simulink model "xpcpid"  (Simulink 7.3)
settings: Solver=FixedStepDiscrete  StartTime=0.0  StopTime=10000  FixedStep=Ts  RelTol=1e-3
values from neighbouring files (symbols this model uses):
  K = 3.86    [Copy_of_benchmark.m]    (also in benchmark.m = 17.85; setpidparam.m = 1)
  mu = 0.1    [Copy_of_benchmark.m]    (also in benchmark.m; setpidparam.m)
  N = 4    [Copy_of_benchmark.m]    (also in benchmark.m = 2; setpidparam.m = 2)
  Td = 0    [Copy_of_benchmark.m]    (also in benchmark.m = 0.2983; setpidparam.m = 0.1)
  theta = [anti_wind_up; anti_bump; Kf]    [Copy_of_benchmark.m]    (also in benchmark.m = [0]; setpidparam.m = 10)
  Ti = 27    [Copy_of_benchmark.m]    (also in benchmark.m = 1.1932; setpidparam.m = 10)
  Ts = 0.02    [Copy_of_benchmark.m]    (also in benchmark.m; setpidparam.m)
  u0 = 4    [Copy_of_benchmark.m]    (also in setpidparam.m = 0)
  ubounds = [0;10]    [Copy_of_benchmark.m]    (also in benchmark.m = [-6;6]; setpidparam.m = [-4;6])
  y0 = 5.5    [Copy_of_benchmark.m]    (also in setpidparam.m = 0)
libraries: xpclib x4, xpcnilib x2
settings Model: Creator=andrecb  LastModifiedBy=petersson  SimulationMode=external  ExtModeTrigDuration=100  BufferReuse=off
settings OptimizationCC: BlockReduction=off  OptimizeBlockIOStorage=off  BufferReuse=off  ExpressionFolding=off  LocalBlockOutputs=off
settings HardwareCC: ProdIntDivRoundTo=Zero  ProdEndianess=LittleEndian  ProdHWDeviceType=Generic->32-bit x86 compatible
settings RTWCC: SystemTargetFile=xpctarget.tlc  TemplateMakefile=xpc_default_tmf  Description=xPC Target  RTWVerbose=off  ProcessScript=xpctarget_make_rtw_hook  RTWCompilerOptimization=On
settings xpcTargetCC: TargetFcnLib=ansi_tfl_table_tmw.mat  TargetFunctionLibrary=ANSI_C  ParMdlRefBuildCompliant=off  PortableWordSizes=off

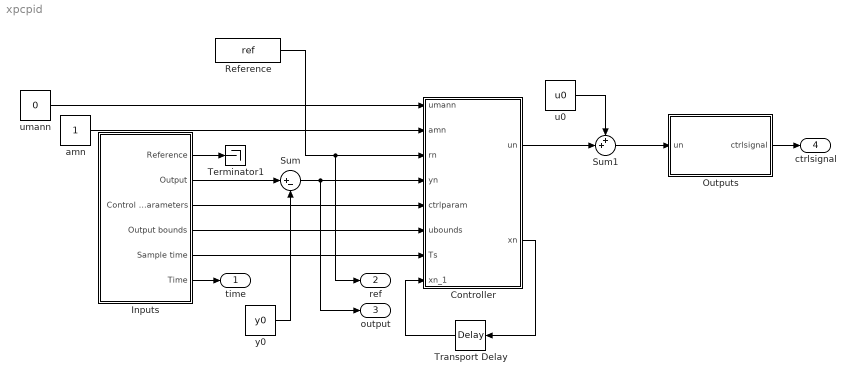
== system xpcpid ==
  Controller : Stateflow chart
  Inputs : Subsystem
  Outputs : Subsystem
  Reference : FromWorkspace  VariableName=ref  SampleTime=Ts
  Sum : Sum  Inputs=|+-  OutDataType=fixdt(1, 16)  OutScaling=2^0
  Sum1 : Sum  Inputs=++|  OutDataType=fixdt(1, 16)  OutScaling=2^0
  Terminator1 : Terminator
  Transport Delay : TransportDelay  DelayTime=Ts  InitialOutput=zeros(N,1)  FixedBuffer=on
  amn : Constant  OutDataType=fixdt(1, 16)  OutScaling=2^0
  u0 : Constant  Value=u0  OutDataType=fixdt(1, 16)  OutScaling=2^0  SampleTime=Ts
  umann : Constant  Value=0  OutDataType=fixdt(1, 16)  OutScaling=2^0
  y0 : Constant  Value=y0  OutDataType=fixdt(1, 16)  OutScaling=2^0  SampleTime=Ts
  time : Outport  SampleTime=Ts  OutDataType=fixdt(1, 16)  OutScaling=2^0
  ref : Outport  Port=2  SampleTime=Ts  OutDataType=fixdt(1, 16)  OutScaling=2^0
  output : Outport  Port=3  SampleTime=Ts  OutDataType=fixdt(1, 16)  OutScaling=2^0
  ctrlsignal : Outport  Port=4  SampleTime=Ts  OutDataType=fixdt(1, 16)  OutScaling=2^0
  wires:
  umann/1 -> Controller/1(umann)
  amn/1 -> Controller/2(amn)
  Inputs/3(Control parameters) -> Controller/5(ctrlparam)
  Controller/2(xn) -> Transport Delay/1
  Transport Delay/1 -> Controller/8(xn_1)
  Inputs/4(Output bounds) -> Controller/6(ubounds)
  Inputs/5(Sample time) -> Controller/7(Ts)
  Inputs/6(Time) -> time/1
  Outputs/1(ctrlsignal) -> ctrlsignal/1
  Controller/1(un) -> Sum1/2
  u0/1 -> Sum1/1
  Sum/1 -> Controller/4(yn), output/1
  Inputs/2(Output) -> Sum/1
  y0/1 -> Sum/2
  Inputs/1(Reference) -> Terminator1/1
  Reference/1 -> ref/1, Controller/3(rn)
  Sum1/1 -> Outputs/1(un)

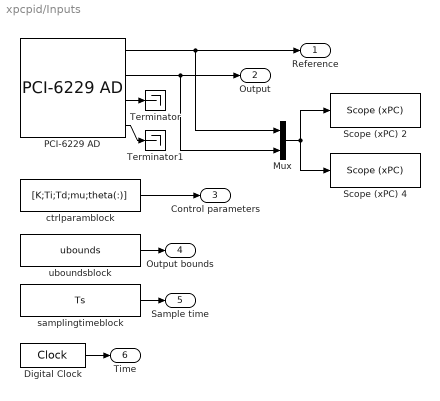
== system xpcpid/Inputs ==
  Digital Clock : DigitalClock  SampleTime=Ts
  Mux : Mux  Inputs=2
  PCI-6229 AD : xpcnilib/A//D/M Series/PCI-6229 AD  channel=[1:4]  range=[10]  coupling=[0]  scantime=5e-6  sampletime=Ts  slot=-1
  Scope (xPC) 2 : xpclib/Misc./Scope (xPC)   SystemSampleTime=-1  scopeno=3  scopetype=Host  autostart=on  viewmode=Graphical rolling  formatstr='%15.6f'  grid=on  ylimits=[0,10]  nosamples=200  noprepostsamples=0  interleave=1  triggermode=FreeRun  triggersignal=1  triggerlevel=0.0  triggerslope=Either  triggerscope=1  triggersample=0  filename=data.dat  mode=Lazy  writesize=512  autorestart=off
  Scope (xPC) 4 : xpclib/Misc./Scope (xPC)   SystemSampleTime=-1  scopeno=4  scopetype=Target  autostart=on  viewmode=Graphical rolling  formatstr='%15.6f'  grid=on  ylimits=[-10,10]  nosamples=200  noprepostsamples=0  interleave=1  triggermode=FreeRun  triggersignal=1  triggerlevel=0.0  triggerslope=Either  triggerscope=1  triggersample=0  filename=data.dat  mode=Lazy  writesize=512  autorestart=off
  Terminator : Terminator
  Terminator1 : Terminator
  ctrlparamblock : Constant  Value=[K;Ti;Td;mu;theta(:)]  OutDataType=fixdt(1, 16)  OutScaling=2^0
  samplingtimeblock : Constant  Value=Ts  OutDataType=fixdt(1, 16)  OutScaling=2^0
  uboundsblock : Constant  Value=ubounds  OutDataType=fixdt(1, 16)  OutScaling=2^0
  Reference : Outport
  Output : Outport  Port=2
  Control parameters : Outport  Port=3
  Output bounds : Outport  Port=4
  Sample time : Outport  Port=5
  Time : Outport  Port=6
  wires:
  PCI-6229 AD/1 -> Mux/1, Reference/1
  PCI-6229 AD/2 -> Mux/2, Output/1
  PCI-6229 AD/3 -> Terminator/1
  PCI-6229 AD/4 -> Terminator1/1
  ctrlparamblock/1 -> Control parameters/1
  uboundsblock/1 -> Output bounds/1
  samplingtimeblock/1 -> Sample time/1
  Digital Clock/1 -> Time/1
  Mux/1 -> Scope (xPC) 4/1, Scope (xPC) 2/1

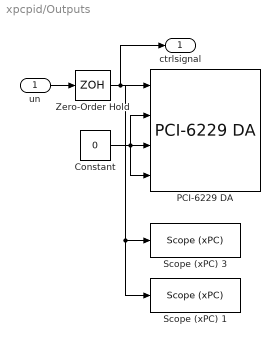
== system xpcpid/Outputs ==
  un : Inport
  Constant : Constant  Value=0  OutDataType=fixdt(1, 16)  OutScaling=2^0
  PCI-6229 DA : xpcnilib/D//A/M Series/PCI-6229 DA  channel=[1:4]  reset=[1]  initValue=[0]  sampletime=Ts  slot=-1
  Scope (xPC) 1 : xpclib/Misc./Scope (xPC)   SystemSampleTime=-1  scopeno=2  scopetype=Target  autostart=on  viewmode=Graphical rolling  formatstr='%15.6f'  grid=on  ylimits=[-10,10]  nosamples=200  noprepostsamples=0  interleave=1  triggermode=FreeRun  triggersignal=1  triggerlevel=0.0  triggerslope=Either  triggerscope=1  triggersample=0  filename=data.dat  mode=Lazy  writesize=512  autorestart=off
  Scope (xPC) 3 : xpclib/Misc./Scope (xPC)   SystemSampleTime=-1  scopeno=1  scopetype=Host  autostart=on  viewmode=Graphical rolling  formatstr='%15.6f'  grid=on  ylimits=[0,10]  nosamples=200  noprepostsamples=0  interleave=1  triggermode=FreeRun  triggersignal=1  triggerlevel=0.0  triggerslope=Either  triggerscope=1  triggersample=0  filename=data.dat  mode=Lazy  writesize=512  autorestart=off
  Zero-Order Hold : ZeroOrderHold  SampleTime=Ts
  ctrlsignal : Outport  SampleTime=Ts  OutDataType=fixdt(1, 16)  OutScaling=2^0
  wires:
  Constant/1 -> PCI-6229 DA/2, PCI-6229 DA/3, PCI-6229 DA/4
  Zero-Order Hold/1 -> PCI-6229 DA/1, ctrlsignal/1, Scope (xPC) 3/1, Scope (xPC) 1/1
  un/1 -> Zero-Order Hold/1

== matlab function Controller ==
  data: umann input double; un output double; amn input double; rn input double; yn input double; ctrlparam input double; ubounds input double; Ts input double; xn_1 input double; xn output double
function [un,xn]=computeux(umann,amn,rn,yn,ctrlparam,ubounds,Ts,xn_1)
K=ctrlparam(1);
Ti=ctrlparam(2);
Td=ctrlparam(3);
mu=ctrlparam(4);
theta=ctrlparam(5:end);

In_1=xn_1(1);
en_1=xn_1(2);
umin=ubounds(1);
umax=ubounds(2);

en=rn-yn;
In=In_1+ K*Ts*en/Ti;
vn=K*en+In+K*Td*(en-en_1)/Ts;
if vn<umin
    un=umin;
elseif vn>umax
    un=umax;
else
    un=vn;
end
xn=[In;en];
